simulink subsystem "calculate_fault_injected_pwm"  (R2024a)
settings: Solver=VariableStepAuto  StartTime=0.0  StopTime=10.0  RelTol=1e-3
settings Model: Creator=UASG  LastModifiedBy=UASG

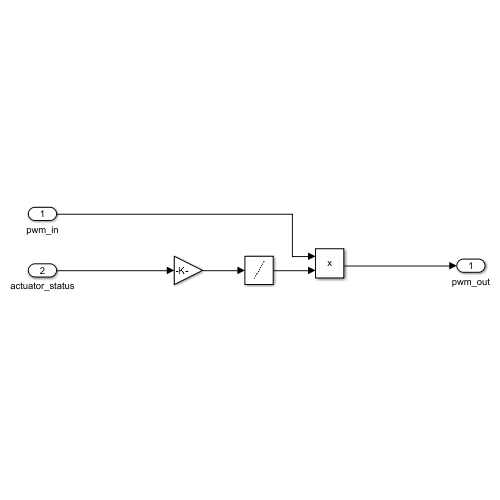
[thumbnail: Simulink's stored preview of the top-level diagram]
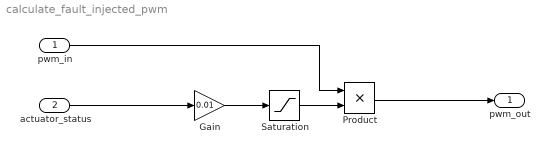
== system calculate_fault_injected_pwm ==
  pwm_in : Inport
  actuator_status : Inport  Port=2
  Gain : Gain  Gain=0.01
  Product : Product
  Saturation : Saturate  UpperLimit=1  LowerLimit=0
  pwm_out : Outport
  wires:
  Product/1 -> pwm_out/1
  actuator_status/1 -> Gain/1
  pwm_in/1 -> Product/1
  Gain/1 -> Saturation/1
  Saturation/1 -> Product/2
